simulink model "Moment_BASA_2014"  (R2014b)
settings: Solver=ode3  SolverMode=SingleTasking  StartTime=0  StopTime=9000  FixedStep=0.01  RelTol=1e-3
settings Model: CovMetricSettings=dwe  CovHtmlReporting=off  covSaveCumulativeToWorkspaceVar=off  CovSaveSingleToWorkspaceVar=off  CovExternalEMLEnable=on  CovSFcnEnable=on  Creator=alexandr.lanin  LastModifiedBy=alexandr.lanin
settings DataIOCC: LimitDataPoints=off  SaveFormat=StructureWithTime
settings DebuggingCC: SolverPrmCheckMsg=none  FrameProcessingCompatibilityMsg=error  SFUnexpectedBacktrackingDiag=error  SFNoUnconditionalDefaultTransitionDiag=error
settings HardwareCC: ProdBitPerPointer=64  ProdLargestAtomicFloat=Float  ProdIntDivRoundTo=Zero  ProdEndianess=LittleEndian  ProdHWDeviceType=Specified
settings ModelReferenceCC: PropagateSignalLabelsOutOfModel=on
settings GRTTargetCC: TargetLangStandard=C99 (ISO)  GeneratePreprocessorConditionals=Use local settings

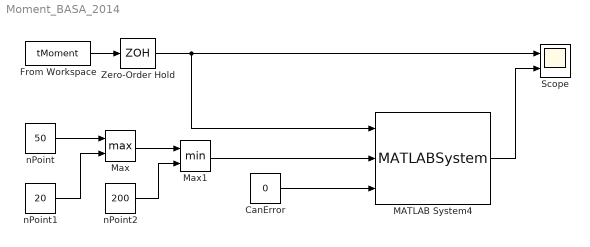
== system Moment_BASA_2014 ==
  CanError : Constant  Value=0
  From Workspace : FromWorkspace  VariableName=tMoment  SampleTime=0
  MATLAB System4 : MATLABSystem  System=CMoment  SimulateUsing=Code generation
      mask Type: CMoment
      mask Display:
      | disp('CMoment');
      | port_label('input',1,'moment');
      | port_label('input',2,'npoint');
      | port_label('input',3,'err');
      | port_label('output',1,'outMoment');
  Max : MinMax  Function=max  Inputs=2
  Max1 : MinMax  Inputs=2
  Scope : Scope  NumInputPorts=2
      settings: TimeRange=auto  MaxDataPoints=5000  SaveToWorkspace=off  SaveName=ScopeData  YMin=125.40523~-5  YMax=280.59954~5  SampleTime=-1
  Zero-Order Hold : ZeroOrderHold  SampleTime=0.01
  nPoint : Constant  Value=50
  nPoint1 : Constant  Value=20
  nPoint2 : Constant  Value=200
  wires:
  CanError/1 -> MATLAB System4/3
  From Workspace/1 -> Zero-Order Hold/1
  Zero-Order Hold/1 -> MATLAB System4/1, Scope/1
  nPoint/1 -> Max/1
  nPoint1/1 -> Max/2
  Max/1 -> Max1/1
  nPoint2/1 -> Max1/2
  Max1/1 -> MATLAB System4/2
  MATLAB System4/1 -> Scope/2
